simulink model "VSI_third_harmonic_injection_PWM"  (R2020b)
settings: Solver=ode45  StartTime=0.0  StopTime=0.1  RelTol=1e-3
InitFcn:
  | clc;
  | f=50;
  | fs=4000;
  | Ts=10e-6;
StopFcn:
  | clc
  | figure(1);
  | plot(sector(:,1),sector(:,2),'-b',ab(:,1),ab(:,2),'-r');
  | axis equal;
  | grid;
  | title('PWM Vetorial');
libraries: powerlib x15, simulink x3
settings Model: Creator=Karim  LastModifiedBy=Karim
settings DataIOCC: ReturnWorkspaceOutputs=off

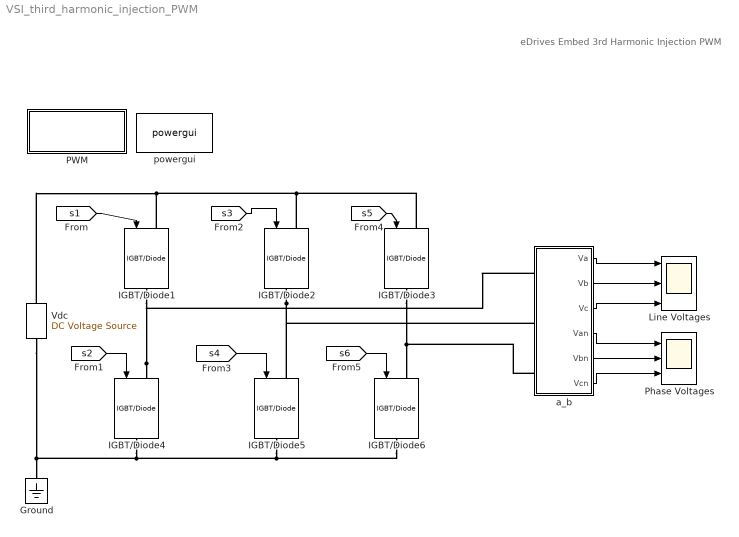
== system VSI_third_harmonic_injection_PWM ==
  note: eDrives Embed
      |
      | 3rd Harmonic Injection PWM
  Ground : powerlib/Elements/Ground  LConnTagsString=a
  IGBT/Diode{1..6} (6 alike) : powerlib/Power Electronics/IGBT//Diode  Ron=1e-3  Rs=1e5  Cs=inf  Measurements=off
  Line Voltages : Scope  NumInputPorts=3
  PWM : Subsystem
  Phase Voltages : Scope  NumInputPorts=3
  Vdc : powerlib/Electrical Sources/DC Voltage Source  Amplitude=400  Measurements=None
  a_b : Subsystem
  powergui : powerlib/powergui  Priority=1  SimulationMode=Continuous  SampleTime=1e-6  frequency=60  Iterations=50  frequencyindice=0  Pbase=100e6  ErrMax=1e-4  UnitsV=kV  UnitsW=MW  buscounter=0  FunctionMessages=off  echomessages=off  EnableUseOfTLC=off  CurrentSourceSwitches=on  DisableSnubberDevices=off  DisableRonSwitches=off  DisableVfSwitches=off  DisplayEquations=off  AutomaticDiscreteSolvers=off  SolverType=Tustin  Interpol=off  ExternalGateDelay=off  methode=off  Ts=0  x0status=blocks  SPID=off  SwTol=0  HookPort=off  NonlinearTolerance=1e-4  nMaxIteration=100  ContinueOnMaxIteration=off  RestoreLinks=warning  ResistiveCurrentMeasurement=off  Frange=[0:2:500]  Ylog=off  Xlog=on  ShowGrid=off  save=off  variable=ZData  structure=Neutral_voltages  ZoomFFT=off  StartTime=0.0  cycles=1  DisplayStyle=1  fundamental=50  FreqAxis=on  MaxFrequency=1000  frequencyindicesteady=1  RmsSteady=1  display=off
  wires:
  [s6] -> IGBT/Diode6/1
  [s5] -> IGBT/Diode3/1
  [s3] -> IGBT/Diode2/1
  [s2] -> IGBT/Diode4/1
  a_b/1(Va) -> Line Voltages/1
  [s4] -> IGBT/Diode5/1
  a_b/5(Vbn) -> Phase Voltages/2
  a_b/2(Vb) -> Line Voltages/2
  a_b/3(Vc) -> Line Voltages/3
  a_b/4(Van) -> Phase Voltages/1
  [s1] -> IGBT/Diode1/1
  a_b/6(Vcn) -> Phase Voltages/3
  connections:
  IGBT/Diode2/RConn1 -- IGBT/Diode5/LConn1 -- a_b/LConn2
  IGBT/Diode4/LConn1 -- IGBT/Diode1/RConn1 -- a_b/LConn1
  IGBT/Diode2/LConn1 -- IGBT/Diode3/LConn1 -- Vdc/RConn1 -- IGBT/Diode1/LConn1
  a_b/LConn3 -- IGBT/Diode3/RConn1 -- IGBT/Diode6/LConn1
  IGBT/Diode6/RConn1 -- IGBT/Diode5/RConn1 -- Ground/LConn1 -- Vdc/LConn1 -- IGBT/Diode4/RConn1

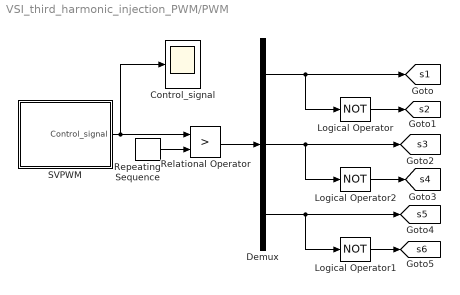
== system VSI_third_harmonic_injection_PWM/PWM ==
  Control_signal : Scope
  Demux : Demux  Outputs=3
  Logical Operator : Logic  Operator=NOT  AllPortsSameDT=off  OutDataTypeStr=boolean
  Logical Operator1 : Logic  Operator=NOT  AllPortsSameDT=off  OutDataTypeStr=boolean
  Logical Operator2 : Logic  Operator=NOT  AllPortsSameDT=off  OutDataTypeStr=boolean
  Relational Operator : RelationalOperator  Operator=>  RndMeth=Nearest
  Repeating Sequence : simulink/Sources/Repeating Sequence  rep_seq_t=[0 0.25/fs 0.5/fs 0.75/fs 1/fs]  rep_seq_y=[1 0 -1 0 1]
  SVPWM : Subsystem
  tag scope: s1=global, s2=global, s3=global, s4=global, s5=global, s6=global
  wires:
  Relational Operator/1 -> Demux/1
  Demux/1 -> [s1], Logical Operator/1
  Demux/2 -> [s3], Logical Operator2/1
  Repeating Sequence/1 -> Relational Operator/2
  Logical Operator/1 -> [s2]
  Logical Operator2/1 -> [s4]
  Logical Operator1/1 -> [s6]
  SVPWM/1(Control_signal) -> Relational Operator/1, Control_signal/1
  Demux/3 -> [s5], Logical Operator1/1

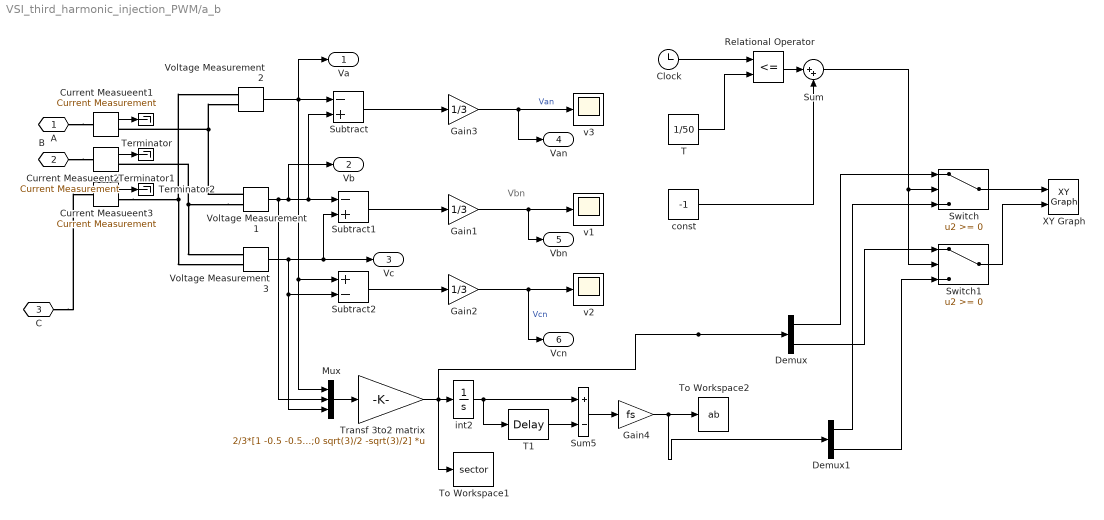
== system VSI_third_harmonic_injection_PWM/a_b ==
  note: Vbn
  Clock : Clock
  Current Measueent1 : powerlib/Measurements/Current Measurement  PhasorSimulation=off  OutputType=Complex  PSBequivalent=0
  Current Measueent2 : powerlib/Measurements/Current Measurement  PhasorSimulation=off  OutputType=Complex  PSBequivalent=0
  Current Measueent3 : powerlib/Measurements/Current Measurement  PhasorSimulation=off  OutputType=Complex  PSBequivalent=0
  Demux : Demux  Outputs=2
  Demux1 : Demux  Outputs=2
  Gain1 : Gain  Gain=1/3
  Gain2 : Gain  Gain=1/3
  Gain3 : Gain  Gain=1/3
  Gain4 : Gain  Gain=fs  SaturateOnIntegerOverflow=on  OutDataTypeStr=Inherit: Same as input  ParamDataTypeStr=Inherit: Same as input
  Mux : Mux  Inputs=3
  Relational Operator : RelationalOperator  Operator=<=  OutDataTypeStr=boolean  RndMeth=Nearest
  Subtract : Sum  Inputs=-+
  Subtract1 : Sum  Inputs=-+
  Subtract2 : Sum  Inputs=+-
  Sum : Sum  Inputs=|++
  Sum5 : Sum  Inputs=+-  InputSameDT=on  SaturateOnIntegerOverflow=on  OutDataTypeStr=Inherit: Same as first input
  Switch : Switch
  Switch1 : Switch
  T : Constant  Value=1/50
  T1 : TransportDelay  DelayTime=1/fs  BufferSize=2048
  Terminator : Terminator
  Terminator1 : Terminator
  Terminator2 : Terminator
  To Workspace1 : ToWorkspace  VariableName=sector  SampleTime=-1
      settings: Decimation=2
  To Workspace2 : ToWorkspace  VariableName=ab  SampleTime=-1
      settings: Decimation=2
  "Transf 3to2 matrix " : Gain  Gain=2/3*[1 -0.5 -0.5;0 sqrt(3)/2 -sqrt(3)/2]  Multiplication=Matrix(K*u)  SaturateOnIntegerOverflow=on  OutDataTypeStr=Inherit: Same as input  ParamDataTypeStr=Inherit: Same as input
  Voltage Measurement1 : powerlib/Measurements/Voltage Measurement  PhasorSimulation=off  OutputType=Complex  PSBequivalent=0
  Voltage Measurement2 : powerlib/Measurements/Voltage Measurement  PhasorSimulation=off  OutputType=Complex  PSBequivalent=0
  Voltage Measurement3 : powerlib/Measurements/Voltage Measurement  PhasorSimulation=off  OutputType=Complex  PSBequivalent=0
  XY Graph : simulink/Sinks/XY Graph  xmin=-500  xmax=500  ymin=-500  ymax=500  st=-1
  const : Constant  Value=-1
  int2 : Integrator
  v1 : Scope
  v2 : Scope
  v3 : Scope
  A : PMIOPort  Side=Left
  B : PMIOPort  Port=2  Side=Left
  C : PMIOPort  Port=3  Side=Left
  Va : Outport
  Vb : Outport  Port=2
  Vc : Outport  Port=3
  Van : Outport  Port=4
  Vbn : Outport  Port=5
  Vcn : Outport  Port=6
  wires:
  Gain2/1 -> v2/1, Vcn/1  "Vcn"
  Subtract2/1 -> Gain2/1
  Gain1/1 -> v1/1, Vbn/1
  Subtract1/1 -> Gain1/1
  Voltage Measurement3/1 -> Subtract1/2, Vc/1, Subtract2/2, Mux/3
  Gain3/1 -> v3/1, Van/1  "Van"
  Subtract/1 -> Gain3/1
  Voltage Measurement1/1 -> Subtract/2, Subtract1/1, Vb/1, Mux/2
  Voltage Measurement2/1 -> Subtract/1, Va/1, Subtract2/1, Mux/1
  Current Measueent1/1 -> Terminator/1
  Current Measueent2/1 -> Terminator1/1
  Current Measueent3/1 -> Terminator2/1
  Mux/1 -> "Transf 3to2 matrix "/1
  T1/1 -> Sum5/2
  int2/1 -> Sum5/1, T1/1
  Sum5/1 -> Gain4/1
  "Transf 3to2 matrix "/1 -> Demux/1, int2/1, To Workspace1/1
  Gain4/1 -> To Workspace2/1, Demux1/1
  Relational Operator/1 -> Sum/1
  Demux/1 -> Switch/1
  Switch/1 -> XY Graph/1
  Switch1/1 -> XY Graph/2
  Demux/2 -> Switch1/1
  Demux1/1 -> Switch/3
  Demux1/2 -> Switch1/3
  Clock/1 -> Relational Operator/1
  T/1 -> Relational Operator/2
  const/1 -> Sum/2
  Sum/1 -> Switch1/2, Switch/2
  connections:
  Voltage Measurement1/LConn1 -- Current Measueent1/RConn1 -- Voltage Measurement2/LConn2
  Voltage Measurement1/LConn2 -- Current Measueent2/RConn1 -- Voltage Measurement3/LConn1
  Current Measueent3/RConn1 -- Voltage Measurement2/LConn1 -- Voltage Measurement3/LConn2
  A/RConn1 -- Current Measueent1/LConn1
  B/RConn1 -- Current Measueent2/LConn1
  C/RConn1 -- Current Measueent3/LConn1

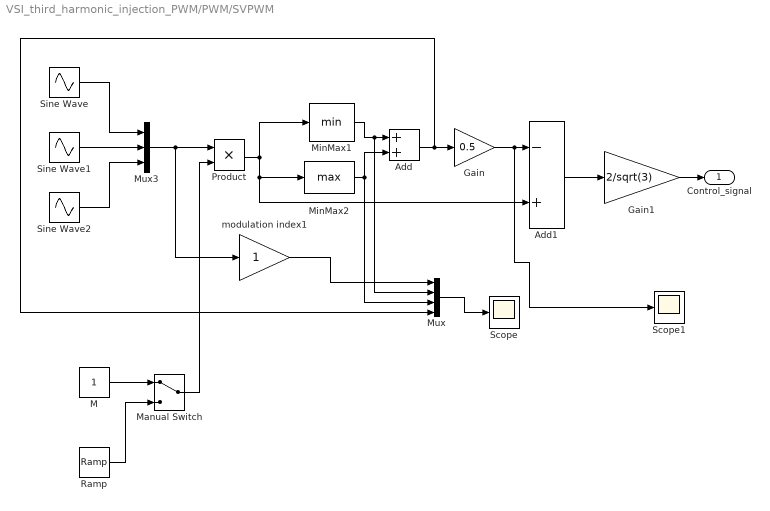
== system VSI_third_harmonic_injection_PWM/PWM/SVPWM ==
  Add : Sum
  Add1 : Sum  Inputs=-+
  Gain : Gain  Gain=0.5
  Gain1 : Gain  Gain=2/sqrt(3)
  M : Constant
  Manual Switch : ManualSwitch
  MinMax1 : MinMax  InputSameDT=on  SaturateOnIntegerOverflow=on
  MinMax2 : MinMax  Function=max  InputSameDT=on  SaturateOnIntegerOverflow=on
  Mux : Mux
  Mux3 : Mux  Inputs=3
  Product : Product
  Ramp : simulink/Sources/Ramp  slope=2  start=0  InitialOutput=0.8
  Scope : Scope
  Scope1 : Scope
  Sine Wave : Sin  Frequency=2*pi*f  Phase=pi/2  SampleTime=0
  Sine Wave1 : Sin  Frequency=2*pi*f  Phase=pi/2-2*pi/3  SampleTime=0
  Sine Wave2 : Sin  Frequency=2*pi*f  Phase=pi/2+ 2*pi/3  SampleTime=0
  modulation index1 : Gain  SaturateOnIntegerOverflow=on  OutDataTypeStr=Inherit: Same as input  ParamDataTypeStr=Inherit: Same as input
  Control_signal : Outport
  wires:
  Sine Wave/1 -> Mux3/1
  Sine Wave1/1 -> Mux3/2
  Sine Wave2/1 -> Mux3/3
  Mux3/1 -> Product/1, modulation index1/1
  Product/1 -> MinMax1/1, Add1/2, MinMax2/1
  MinMax2/1 -> Mux/3, Add/2
  Add/1 -> Mux/4, Gain/1
  Gain/1 -> Scope1/1, Add1/1
  Add1/1 -> Gain1/1
  Gain1/1 -> Control_signal/1
  MinMax1/1 -> Mux/2, Add/1
  Mux/1 -> Scope/1
  modulation index1/1 -> Mux/1
  M/1 -> Manual Switch/1
  Ramp/1 -> Manual Switch/2
  Manual Switch/1 -> Product/2
